simulink library "DQN_Lib (conflicted copy 2023-11-25 155310)"  (R2023b)
settings: Solver=VariableStepAuto  StartTime=0.0  StopTime=10.0  RelTol=1e-3
undefined symbols (not defined in the file): FreqRad, HrmOrd, Init, La, N, R, Ra, TimeStep, Ts, Ts_dqn, Ws
libraries: $bdroot x4, spsMeanVariableFrequencyLib x4, eeTransforms x3, spsabctodq0Lib x2, spsAlphaBetaZerotodq0Lib x1
(part 8 of 8)

== matlab function DQN_Lib (conflicted copy 2023-11-25 155310)/BACKUP/Gain_DQNc_Mat1 ==
  data: Xpnz input; Ypnz output; Rabc parameter; chkInv parameter; HRM parameter
function Ypnz  = Gain_Mat2(Xpnz, Rabc, chkInv, HRM)
    persistent Rpnz;
    %persistent nrInp;
    % persistent nrOut;

    mrows = size(Rabc,1)/3; %signal size
    mcols = size(Rabc,2)/3; %signal size

    nrInp = size(Rabc,1);

    Ypnz = complex(zeros(nrInp, HRM+1));


    if(isempty(Rpnz)) 

        Rpnz = complex(zeros(3*mrows,3*mcols));
        a = -0.5+0.866i;
        a2 = -0.5-0.866i;
        Sas = [1,a,a2;1,a2,a;1,1,1]/3;
        %Ssa = eye(3)/(Sas);
        %nrInp = size(Xpnz,1) / 3;

        for i = 1 : mrows
            for j = 1 : mcols
                Rpnz((1:3) + (i-1)*3,(1:3) + (j-1)*3) = Sas*Rabc((1:3) + (i-1)*3,(1:3) + (j-1)*3)/Sas;
            end
        end

        if(chkInv)
            %Rpnz((1:3) + (i-1)*3,(1:3) + (j-1)*3) = eye(3)/Rpnz((1:3) + (i-1)*3,(1:3) + (j-1)*3);
            Rpnz = eye(3*mrows,3*mcols)/Rpnz;
        end

    end




    
    Ypnz = Rpnz*Xpnz;

end

== matlab function DQN_Lib (conflicted copy 2023-11-25 155310)/Gain_DQNc_Mat ==
  data: Xpnz input; Ypnz output; Rabc parameter; chkInv parameter; HRM parameter
function Ypnz  = Gain_Mat2(Xpnz, Rabc, chkInv, HRM)
    persistent Rpnz;
    %persistent nrInp;
    persistent nrOut;

    mrows = size(Rabc,1)/3; %signal size
    mcols = size(Rabc,2)/3; %signal size

    nrInp = size(Rabc,1);

    % Ypnz = complex(zeros(nrInp, HRM+1));


    if(isempty(Rpnz)) 

        Rpnz = complex(zeros(3*mrows,3*mcols));
        a = -0.5+0.866i;
        a2 = -0.5-0.866i;
        Sas = [1,a,a2;1,a2,a;1,1,1]/3;
        %Ssa = eye(3)/(Sas);
        %nrInp = size(Xpnz,1) / 3;

        for i = 1 : mrows
            for j = 1 : mcols
                Rpnz((1:3) + (i-1)*3,(1:3) + (j-1)*3) = Sas*Rabc((1:3) + (i-1)*3,(1:3) + (j-1)*3)/Sas;
            end
        end

        if(chkInv)
            %Rpnz((1:3) + (i-1)*3,(1:3) + (j-1)*3) = eye(3)/Rpnz((1:3) + (i-1)*3,(1:3) + (j-1)*3);
            Rpnz = eye(3*mrows,3*mcols)/Rpnz;
        end

    end




    
    Ypnz = Rpnz*Xpnz;

end

== matlab function DQN_Lib (conflicted copy 2023-11-25 155310)/Int_DQNc_Mat ==
  settings: updateMethod=DISCRETE
  data: Xpnz input; N parameter; dt parameter; w parameter; InitInt parameter; Zpnz output; R parameter; iL parameter; swFeed parameter
function Zpnz    = Int_DQN_Mat(Xpnz, N, dt, w, InitInt, R, iL, swFeed)


    nrSig = size(Xpnz,1)/3;
    Zpnz = complex(zeros(nrSig*3,N+1));

    persistent Zpnz_old;
    persistent Xpnz_old;
    persistent Krl1;
    persistent Krl2;
    persistent dt2;
        
    if(isempty(Zpnz_old)) 
    


        
        % if(~isempty(InitInt))
        % Zpnz_old(:,1) = Sas * InitInt;
        % end


        Zpnz_old = complex(zeros(nrSig*3,N+1));
        Xpnz_old = complex(zeros(nrSig*3,N+1));
        dt2 = dt/2;

        if(swFeed)
            mrows = size(R,1)/3; %signal size
            mcols = size(R,2)/3; %signal size

            szMatR = size(R,1);
            szMatiL = size(iL,1);

            if(szMatiL ~= szMatR || size(R,1) ~= size(R,2) || size(iL,1) ~= size(iL,2))
                error('[Int_DQN_Mat/swFeedback] check matrix sizes!');
            end
    
            Rpnz = complex(zeros(3*mrows,3*mcols));
            iLpnz = complex(zeros(3*mrows,3*mcols));

            a = -0.5+0.866i;
            a2 = -0.5-0.866i;
            Sas = [1,a,a2;1,a2,a;1,1,1]/3;
    
            for i = 1 : mrows
                for j = 1 : mcols
                     Rpnz((1:3) + (i-1)*3,(1:3) + (j-1)*3) = Sas*R((1:3) + (i-1)*3,(1:3) + (j-1)*3)/Sas;
                    iLpnz((1:3) + (i-1)*3,(1:3) + (j-1)*3) = Sas*iL((1:3) + (i-1)*3,(1:3) + (j-1)*3)/Sas;
                end
            end

            Rpnz  = diag(diag(real(Rpnz)));
            iLpnz = diag(diag(real(iLpnz)));

            Krl1 = (iLpnz/(eye(szMatR)+dt2*Rpnz*iLpnz));
            Krl2 = (eye(szMatR)-dt2*Rpnz*iLpnz)/(eye(szMatR)+dt2*Rpnz*iLpnz);
        else
            Krl1 = 1;
            Krl2 = 1;
        end
            
    end

    if(swFeed)
        Zpnz(:,1) = Krl1*dt2*(Xpnz(:,1)+Xpnz_old(:,1))+Krl2*Zpnz_old(:,1);
    else
        Zpnz(:,1) = dt2*(Xpnz(:,1)+Xpnz_old(:,1))+Zpnz_old(:,1);
    end

    Xpnz_old(:,1) = Xpnz(:,1);
    Zpnz_old(:,1) = Zpnz(:,1);

    for i = 1 : N
        if(N>0)
            wn =  i * w; 
            wndt2 = wn*dt2;

            A = 2*dt2/(1+wndt2^2);
            B = (1-wndt2^2)/(1+wndt2^2);

            if(swFeed)

                Zpnz(:,i+1) =      Krl1*A*(real(Xpnz(:,i+1))+wndt2*imag(Xpnz(:,i+1)))+Krl2*(B*real(Zpnz_old(:,i+1))+A*wn*imag(Zpnz_old(:,i+1))) ...
                             + 1i*(Krl1*A*(imag(Xpnz(:,i+1))-wndt2*real(Xpnz(:,i+1)))+Krl2*(B*imag(Zpnz_old(:,i+1))-A*wn*real(Zpnz_old(:,i+1))));
            else
                Zpnz(:,i+1) =      A*(real(Xpnz(:,i+1))+wndt2*imag(Xpnz(:,i+1)))+(B*real(Zpnz_old(:,i+1))+A*wn*imag(Zpnz_old(:,i+1))) ...
                             + 1i*(A*(imag(Xpnz(:,i+1))-wndt2*real(Xpnz(:,i+1)))+(B*imag(Zpnz_old(:,i+1))-A*wn*real(Zpnz_old(:,i+1))));
            end

            Zpnz_old(:,i+1) = Zpnz(:,i+1);

        end
    end


end

== matlab function DQN_Lib (conflicted copy 2023-11-25 155310)/Int_DQN/Int_d_2N_2 ==
  settings: updateMethod=DISCRETE
  data: Zdp output; Xdp input; Xdn input; Xdz input; Xqp input; Xqn input; Xqz input; Zdn output; N parameter; dt parameter; w parameter; EMT parameter; Zdz output; Zqp output; Zqn output; Zqz output; InitInt parameter; chkHrmLst parameter; HrmLst parameter
function [Zdp,Zdn,Zdz,Zqp,Zqn,Zqz]  = IntDQN(Xdp, Xdn, Xdz, Xqp, Xqn, Xqz, N, dt, w, EMT, InitInt, chkHrmLst, HrmLst)

    persistent Zdc_old;    
    persistent Xdc_old;   
    persistent Zdp_old;    
    persistent Zqp_old;    
    persistent Zdn_old;    
    persistent Zqn_old;    
    persistent Zdz_old;    
    persistent Zqz_old;  
       
    persistent HrmLst2;
    persistent dt2;
    persistent range;
    
    Xdc = zeros(6,1);
    Zdc = zeros(6,1);
    
    Xdc(1) = Xdp(1);
    Xdc(2) = Xdn(1);
    Xdc(3) = Xdz(1);
    Xdc(4) = Xqp(1);
    Xdc(5) = Xqn(1);
    Xdc(6) = Xqz(1);

    Xdp = [Xdp(2:end); zeros(N-numel(Xdp)+1,1)];
    Xqp = [Xqp(2:end); zeros(N-numel(Xqp)+1,1)];
    Xdn = [Xdn(2:end); zeros(N-numel(Xdn)+1,1)];
    Xqn = [Xqn(2:end); zeros(N-numel(Xqn)+1,1)];
    Xdz = [Xdz(2:end); zeros(N-numel(Xdz)+1,1)];
    Xqz = [Xqz(2:end); zeros(N-numel(Xqz)+1,1)];
       
    Zdp = zeros(N+1,1);
    Zdn = zeros(N+1,1);
    Zqp = zeros(N+1,1);
    Zqn = zeros(N+1,1);
    Zdz = zeros(N+1,1);
    Zqz = zeros(N+1,1);
    
    if(isempty(Zdc_old)) 
        Zdc_old  = InitInt';
        Xdc_old  = zeros(6,1);
        
        Zdp_old  = zeros(N,1); Zdp_old(1) = InitInt(1);
        Zdn_old  = zeros(N,1); Zdn_old(1) = InitInt(2);
        Zdz_old  = zeros(N,1); Zdz_old(1) = InitInt(3);
        Zqp_old  = zeros(N,1); Zqp_old(1) = InitInt(4);
        Zqn_old  = zeros(N,1); Zqn_old(1) = InitInt(5);
        Zqz_old  = zeros(N,1); Zqz_old(1) = InitInt(6);
        
        if(isempty(HrmLst2))            
            HrmLst2 = HrmLst;
            HrmLst2(HrmLst2==0) = [];
        end
        dt2 = dt/2;  
        
        if(chkHrmLst)
            range = numel(HrmLst2);
        else
            range = N; 
        end
        
    end

    
    
    Zdc(:) = dt2*(Xdc(:)+Xdc_old(:))+Zdc_old(:);
    Zdc_old = Zdc;
    Xdc_old = Xdc;


    if(N>0)
        A = 0;
        

        
        i = 1;

        for g = 1 : range
            
            if(chkHrmLst)
                if(HrmLst2(g)>0)
                    i = HrmLst2(g);
                end
            else
                i = g; 
            end
            
            
            wn =  i * w; 

            if(EMT)

                A = 2/(1+(dt2*wn)^2);
                %A = 1/(1+(dt2*wn)^2);

                wndt2 = wn*dt2;

                %%% POS %%%
                K1 = dt2*(2*Xdp(i)+Zqp_old(i)*wn) + Zdp_old(i);
                K2 = dt2*(2*Xqp(i)-Zdp_old(i)*wn) + Zqp_old(i);

                Zdp(i) = A*( K1 + wndt2*K2)/2;
                Zqp(i) = A*( K2 - wndt2*K1)/2;
                %Zdp(i) = A*( K1 + wndt2*K2);
                %Zqp(i) = A*( K2 - wndt2*K1);

                Zdp_old(i) = Zdp(i);
                Zqp_old(i) = Zqp(i); 

                %%% NEG %%%
                K1 = dt2*(2*Xdn(i)-Zqn_old(i)*wn) + Zdn_old(i);
                K2 = dt2*(2*Xqn(i)+Zdn_old(i)*wn) + Zqn_old(i);

                Zdn(i) = A*( K1 - wndt2*K2)/2;
                Zqn(i) = A*( K2 + wndt2*K1)/2;
                %Zdn(i) = A*( K1 - wndt2*K2);
                %Zqn(i) = A*( K2 + wndt2*K1);

                Zdn_old(i) = Zdn(i);
                Zqn_old(i) = Zqn(i);

                %%% ZERO %%%
                K1 = dt2*(2*Xdz(i)+Zqz_old(i)*wn) + Zdz_old(i);
                K2 = dt2*(2*Xqz(i)-Zdz_old(i)*wn) + Zqz_old(i);

                Zdz(i) = A*( K1 + wndt2*K2)/2;
                Zqz(i) = A*( K2 - wndt2*K1)/2;
                %Zdz(i) = A*( K1 + wndt2*K2);
                %Zqz(i) = A*( K2 - wndt2*K1);

                Zdz_old(i) = Zdz(i);
                Zqz_old(i) = Zqz(i);

            else
    
                Tad_p2 = (2/3)*[sin(0) sin(0-2*pi/3) sin(0+2*pi/3);  
                               cos(0) cos(0-2*pi/3) cos(0+2*pi/3);];

                Tad_z2 = (1/3)*[sin(0) sin(0) sin(0);  
                               cos(0) cos(0) cos(0);];

                Ta_dqn = [Tad_p2(1,:); Tad_p2(1,:); Tad_z2(1,:); Tad_p2(2,:); Tad_p2(2,:); Tad_z2(2,:)];

                Zdp(i) = (Xqp(i))*(1/(wn));
                Zqp(i) = (Xdp(i))*(-1/(wn)); 

                Zdn(i) = (Xqn(i))*(-1/(wn));
                Zqn(i) = (Xdn(i))*(1/(wn)); 

                Zdz(i) = (Xqz(i))*(1/(wn));
                Zqz(i) = (Xdz(i))*(-1/(wn));
                

                sT = sin(2*pi/3);
                cT = cos(2*pi/3);
%                 Zdc([1,4, 3]) = Zdc([1,4, 3])-Tad_p*[Zqp(i);-sT*Zdp(i)+cT*Zqp(i);sT*Zdp(i)+cT*Zqp(i)];
%                 Zdc([1,4, 3]) = Zdc([1,4, 3])-Tad_p*[Zqn(i);-sT*Zdn(i)+cT*Zqn(i);sT*Zdn(i)+cT*Zqn(i)];
%                 Zdc([1,4, 3]) = Zdc([1,4, 3])-Tad_p*[Zqz(i); Zqz(i)             ;Zqz(i)];

                Zdc = Zdc-Ta_dqn*[Zqp(i);-sT*Zdp(i)+cT*Zqp(i);sT*Zdp(i)+cT*Zqp(i)];
                Zdc = Zdc-Ta_dqn*[Zqn(i);-sT*Zdn(i)+cT*Zqn(i);sT*Zdn(i)+cT*Zqn(i)];
                Zdc = Zdc-Ta_dqn*[Zqz(i); Zqz(i)             ;Zqz(i)];

            end
            

        end

        Zdp(2:end) = Zdp(1:end-1);
        Zdn(2:end) = Zdn(1:end-1);
        Zdz(2:end) = Zdz(1:end-1);
        Zqp(2:end) = Zqp(1:end-1);
        Zqn(2:end) = Zqn(1:end-1);
        Zqz(2:end) = Zqz(1:end-1);


    end
    
    Zdp(1)     = Zdc(1);
    Zdn(1)     = Zdc(2);
    Zdz(1)     = Zdc(3);
    Zqp(1)     = Zdc(4);
    Zqn(1)     = Zdc(5);
    Zqz(1)     = Zdc(6);
end

== matlab function DQN_Lib (conflicted copy 2023-11-25 155310)/DQN2abc/DQn->ABC19 ==
  data: Xdp input; Xdn input; Xdz input; Xqp input; Xqn input; Xqz input; th input; abc output; N parameter
%function abc = Mult(Z0,Zdp,Zqp,Zdn,Zqn,Zdz,Zqz,th, N)
function abc = dqn2abc(Xdp,Xdn,Xdz,Xqp,Xqn,Xqz,th,N)

    %Xdc = zeros(1,6);
    Xdc = zeros(6,1);

    persistent Tda_p2;
    persistent Tdqn_a;
    
    if(isempty(Tda_p2)) 
        Tda_p2 = [-0           1     1;
                 -sqrt(3/4)  -0.5   1;
                  sqrt(3/4)  -0.5   1;];
                Tdqn_a = zeros(3,6);
                Tdqn_a = [Tda_p2(:,1)  Tda_p2(:,1)  0*Tda_p2(:,3)  Tda_p2(:,2)  Tda_p2(:,2)  2*Tda_p2(:,3)]/2;
    end


    Xdc(1) = Xdp(1);
    Xdc(2) = Xdn(1);
    Xdc(3) = Xdz(1);
    Xdc(4) = Xqp(1);
    Xdc(5) = Xqn(1);
    Xdc(6) = Xqz(1);

    abc = Tdqn_a*Xdc;

    abc3p = [0;0;0];
    abc3n = [0;0;0];
    abc1p = [0;0;0];
 

    for i = 1 : N

        Tda_p = [sin(i*th)          cos(i*th);
                 sin(i*th-2*pi/3)   cos(i*th-2*pi/3);
                 sin(i*th+2*pi/3)   cos(i*th+2*pi/3)];
        Tda_n = [sin(-i*th)         cos(-i*th);
                 sin(-i*th-2*pi/3)  cos(-i*th-2*pi/3);
                 sin(-i*th+2*pi/3)  cos(-i*th+2*pi/3)];
        Tda_z = [sin(i*th)          cos(i*th);
                 sin(i*th-0*pi/3)   cos(i*th-0*pi/3);
                 sin(i*th+0*pi/3)   cos(i*th+0*pi/3)];

        abc3p = abc3p + Tda_p*[Xdp(i+1);Xqp(i+1)];
        abc3n = abc3n + Tda_n*[Xdn(i+1);Xqn(i+1)];
        abc1p = abc1p + Tda_z*[Xdz(i+1);Xqz(i+1)];  

    end

    abc = abc+abc3p+abc3n+abc1p;%+abc1n;

== matlab function DQN_Lib (conflicted copy 2023-11-25 155310)/Add_DQN/MATLAB Function1 ==
  data: Xdp input; Xdn input; Xdz input; Xqp input; Xqn input; Xqz input; Ydp input; Ydn input; Ydz input; Yqp input; Yqn input; Yqz input; Zdp output; Zdn output; Zdz output; Zqp output; Zqn output; Zqz output; N parameter; chkHrmLst parameter; HrmLst parameter
function [Zdp,Zdn,Zdz,Zqp,Zqn,Zqz]  = SumDQN(Xdp, Xdn, Xdz, Xqp, Xqn, Xqz, Ydp, Ydn, Ydz, Yqp, Yqn, Yqz, N, chkHrmLst, HrmLst)
%function [Zdc,Zdp,Zqp,Zdn,Zqn,Zdz,Zqz]  = SumDQN(Xdc, Xdp, Xdn, Xdz, Xqp, Xqn, Xqz, Ydc, Ydp, Ydn, Ydz, Yqp, Yqn, Yqz, N)

    Xdp = [Xdp(1:end); zeros(N+1-numel(Xdp),1)];
    Ydp = [Ydp(1:end); zeros(N+1-numel(Ydp),1)];
    Xqp = [Xqp(1:end); zeros(N+1-numel(Xqp),1)];
    Yqp = [Yqp(1:end); zeros(N+1-numel(Yqp),1)];
      
    Xdn = [Xdn(1:end); zeros(N+1-numel(Xdn),1)];
    Ydn = [Ydn(1:end); zeros(N+1-numel(Ydn),1)];
    Xqn = [Xqn(1:end); zeros(N+1-numel(Xqn),1)];
    Yqn = [Yqn(1:end); zeros(N+1-numel(Yqn),1)];
    
    Xdz = [Xdz(1:end); zeros(N+1-numel(Xdz),1)];
    Ydz = [Ydz(1:end); zeros(N+1-numel(Ydz),1)];
    Xqz = [Xqz(1:end); zeros(N+1-numel(Xqz),1)];
    Yqz = [Yqz(1:end); zeros(N+1-numel(Yqz),1)];
       
    Zdp = zeros(N+1,1);
    Zdn = zeros(N+1,1);
    Zqp = zeros(N+1,1);
    Zqn = zeros(N+1,1);
    Zdz = zeros(N+1,1);
    Zqz = zeros(N+1,1);
    
    persistent range;
    
    if(isempty(range))        
        if(chkHrmLst)
            range = numel(HrmLst);
        else
            range = N+1; 
        end
    end
         
    h = 1;
    
    for i = 1 : range
        
        if(chkHrmLst)
            if(HrmLst(i)>0)
                h = HrmLst(i)+1;
            end
        else
            h = i; 
        end
        
        Zdp(h) = Xdp(h)+Ydp(h);
        Zdn(h) = Xdn(h)+Ydn(h);
        Zqp(h) = Xqp(h)+Yqp(h);
        Zqn(h) = Xqn(h)+Yqn(h);
        Zdz(h) = Xdz(h)+Ydz(h);
        Zqz(h) = Xqz(h)+Yqz(h);
    end
end
